simulink model "Traffic_Lights"  (R2020b)
settings: Solver=VariableStepAuto  StartTime=0.0  StopTime=10.0  RelTol=1e-3
undefined symbols (not defined in the file): Chart, traffic_stateflow
settings Model: EnablePacing=on  PacingRate=0.450000  Creator=lenovo  LastModifiedBy=lenovo

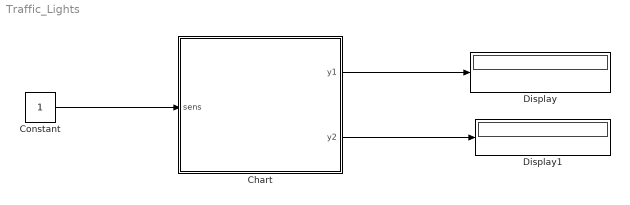
== system Traffic_Lights ==
  Chart : Stateflow chart  AncestorBlock=traffic_stateflow/Chart  TreatAsAtomicUnit=on
  Constant : Constant
  Display : Display
  Display1 : Display
  wires:
  Chart/1(y1) -> Display/1
  Chart/2(y2) -> Display1/1
  Constant/1 -> Chart/1(sens)

== stateflow chart Traffic_Lights/Chart ==
  state stop
    y1='RED';
    y2='GREEN';
  state stopForTraffic
    y1='RED';
    y2='GREEN';
  state StopTorGo
    y1='RED';
    y2='YELLOW';
  state GoToStop
    y1='YELLOW';
    y2='RED';
  state Go
    y1='GREEN';
    y2='RED';
  (default) -> stop
  stop -> stopForTraffic : after(20,tick)
  stopForTraffic -> StopTorGo : [sens==1]
  GoToStop -> stop : after(3,tick)
  StopTorGo -> Go : after(3,tick)
  Go -> GoToStop : after(10,tick)
  data: sens input; y1 output stringtype(8); y2 output stringtype(8); GREEN constant double; RED constant double; YELLOW constant double
